simulink model "projetoRobotica"  (R2015a)
settings: Solver=ode1  StartTime=0.0  StopTime=inf  FixedStep=0.001  RelTol=1e-3
undefined symbols (not defined in the file or in its folder): qc_get_step_size
libraries: simulink x37, simulink_extras x12, quarc_library x8, instrumentlib x1
settings Model: SimulationMode=external  ExtModeTrigDuration=10000  Creator=CFulford  LastModifiedBy=RAS
settings SolverCC: PositivePriorityOrder=on
settings DataIOCC: LimitDataPoints=off  MaxDataPoints=10000  SignalLoggingSaveFormat=ModelDataLogs
settings OptimizationCC: ExpressionDepthLimit=2147483647  InitFltsAndDblsToZero=on
settings DebuggingCC: AlgebraicLoopMsg=none  SaveWithParameterizedLinksMsg=none  UnderspecifiedInitializationDetection=Classic  MergeDetectMultiDrivingBlocksExec=none  SolverPrmCheckMsg=warning  FcnCallInpInsideContextMsg=UseLocalSettings  StateNameClashWarn=warning
settings SFSimCC: SimParseCustomCode=off
settings RTWCC: SystemTargetFile=quarc_win64.tlc  TemplateMakefile=quarc_default_tmf  Description=QUARC Win64 Target
settings STFCustomTargetCC: TargetLibSuffix=.lib  TargetPreCompLibLocation=C:\PROGRA~3\QUARC\lib\2015a\win64\release  GenerateSampleERTMain=off  ConcurrentExecutionCompliant=on  GeneratePreprocessorConditionals=Disable all  CombineOutputUpdateFcns=on  ERTCustomFileBanners=off  SupportNonInlinedSFcns=on  SupportVariableSizeSignals=off  MATLABClassNameForMDSCustomization=Simulink.SoftwareTarget.GRTCustomization  CPPClassGenCompliant=on  SystemTargetFile=quarc_win64.tlc
settings GRTTargetCC: TargetPreCompLibLocation=C:\PROGRA~3\QUARC\lib\2015a\win64\release  ParMdlRefBuildCompliant=off  CompOptLevelCompliant=off  MatFileLogging=off  ExtMode=on  ExtModeMexFile=quarc_comm

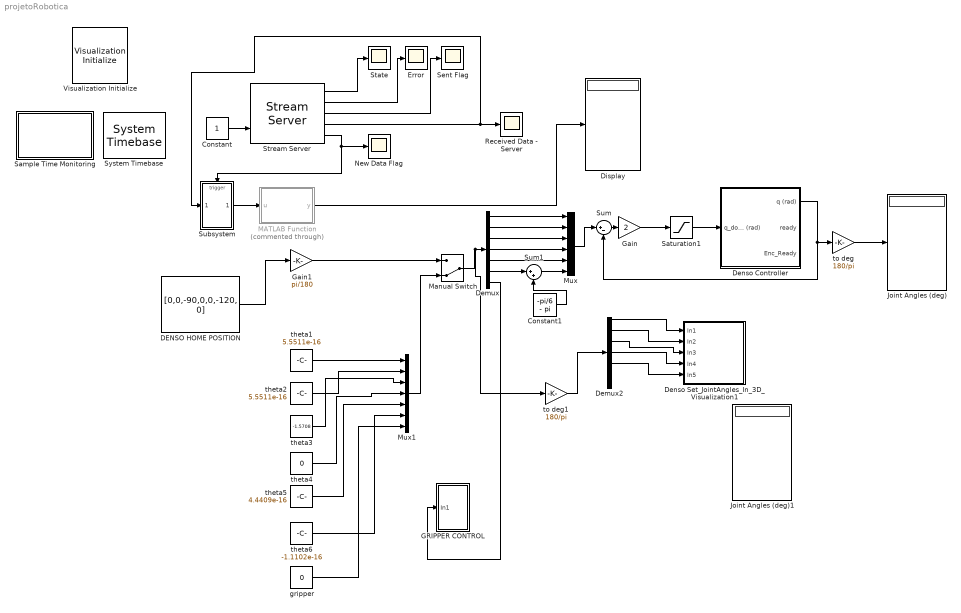
== system projetoRobotica ==
  Constant : Constant
  Constant1 : Constant  Value=-pi/6 - pi
  DENSO HOME POSITION : Constant  Value=[0,0,-90,0,0,-120, 0]  OutDataTypeStr=double  SampleTime=-1
  Demux : Demux  Outputs=7
  Demux2 : Demux  Outputs=7
  Denso Set_JointAngles_In_3D_Visualization1 : Subsystem
  Denso Controller : Subsystem
  Display : Display
  Error : Scope
      settings: SaveName=ScopeData6
  GRIPPER CONTROL : Subsystem
  Gain : Gain  Gain=2
  Gain1 : Gain  Gain=pi/180
  Joint Angles (deg) : Display
      settings: Decimation=100
  Joint Angles (deg)1 : Display
      settings: Decimation=100
  MATLAB Function : MATLAB Function  Commented=through  TreatAsAtomicUnit=on
  Manual Switch : ManualSwitch  CurrentSetting=0
  Mux : Mux  Inputs=6
  Mux1 : Mux  Inputs=7
  New Data Flag : Scope
      settings: SaveName=ScopeData7
  Received Data - Server : Scope
      settings: YMin=-0.2  YMax=1.2  SaveName=ScopeData8
  Sample Time Monitoring : Subsystem
  Saturation1 : Saturate  UpperLimit=200*pi/180  LowerLimit=-200*pi/180  OutDataTypeStr=double
  Sent Flag : Scope
      settings: SaveName=ScopeData5
  State : Scope
      settings: YMin=0  YMax=2
  Stream Server : quarc_library/Communications/Basic/Stream Server  uri_source=Specify via dialog (do not evaluate)  uri=tcpip://localhost:17001  apply_uri_to_all_configs=on  send_buffer_size=1460  receive_buffer_size=1460  byte_order=little endian (Intel - LSB first)  optimization=Minimum latency  implementation=Use non-blocking I/O  send_options=Send most recent data  receive_options=Receive most recent data  send_fifo_size=1000  receive_fifo_size=1000  send_priority=0  receive_priority=0  default_value=[0, 0, -pi/2, 0, 0, 0, 0]  send_dimensions=off  receive_dimensions=off  max_dimensions=-1  sample_time=qc_get_step_size  active=on  data_type=double  type_expr=BusObject
      settings: AttributesFormatString="\"tcpip://localhost:17001\""
  Subsystem : Subsystem
  Sum : Sum  Inputs=|+-
  Sum1 : Sum  Inputs=|++
  System Timebase : quarc_library/Advanced/Timing/System Timebase  stop_on_overrun=off
  Visualization Initialize : quarc_library/User Interface/Visualization/Visualization Initialize  object_name=kinect_direct_kinematics_3_angles_3D_Visualization  scene_file=kinect_direct_kinematics_3_angles_3D_Visualization.xml  uri={'normal','';'Configuration','shmem://%m:2';}  apply_uri_to_all_configs=off  server_send_size=1000000  server_receive_size=1000  derive_from_server=on  client_send_size=1000  client_receive_size=1000000  variables=[ 31 41 51 61 71 ]  initial_values=single([ 0 0 0 0 0 0 0 -1.5708 0 0 0 0 0 0 0 ])  open_on_start=on  close_on_stop=on
      settings: AttributesFormatString=%<object_name>
  gripper : Constant  Value=0
  theta1 : Constant  Value=5.5511e-16
  theta2 : Constant  Value=5.5511e-16
  theta3 : Constant  Value=-1.5708
  theta4 : Constant  Value=0
  theta5 : Constant  Value=4.4409e-16
  theta6 : Constant  Value=-1.1102e-16
  to deg : Gain  Gain=180/pi  OutDataTypeStr=single
  to deg1 : Gain  Gain=180/pi  ParamDataTypeStr=double  OutDataTypeStr=single
  wires:
  Stream Server/1 -> State/1
  Stream Server/2 -> Error/1
  Constant/1 -> Stream Server/2
  Stream Server/3 -> Sent Flag/1
  Stream Server/5 -> New Data Flag/1, Subsystem/Trigger
  Stream Server/4 -> Subsystem/1(In1), Received Data - Server/1
  to deg/1 -> Joint Angles (deg)/1
  Sum/1 -> Gain/1
  Gain/1 -> Saturation1/1
  Denso Controller/1(q (rad)) -> to deg/1, Sum/2
  Saturation1/1 -> Denso Controller/1(q_dot_cmd (rad))
  Subsystem/1(Out1) -> MATLAB Function/1(u)
  DENSO HOME POSITION/1 -> Gain1/1
  Demux2/5 -> Denso Set_JointAngles_In_3D_Visualization1/5(In5)
  Demux2/4 -> Denso Set_JointAngles_In_3D_Visualization1/4(In4)
  Demux2/2 -> Denso Set_JointAngles_In_3D_Visualization1/2(In2)
  Demux2/3 -> Denso Set_JointAngles_In_3D_Visualization1/3(In3)
  Demux2/1 -> Denso Set_JointAngles_In_3D_Visualization1/1(In1)
  to deg1/1 -> Demux2/1
  Manual Switch/1 -> to deg1/1, Demux/1
  Mux/1 -> Sum/1
  Demux/1 -> Mux/1
  Demux/2 -> Mux/2
  Demux/3 -> Mux/3
  Demux/4 -> Mux/4
  Demux/5 -> Mux/5
  Demux/7 -> GRIPPER CONTROL/1(In1)
  MATLAB Function/1(y) -> Display/1
  Demux/6 -> Sum1/1
  Sum1/1 -> Mux/6
  Constant1/1 -> Sum1/2
  theta1/1 -> Mux1/1
  theta2/1 -> Mux1/2
  theta4/1 -> Mux1/4
  theta5/1 -> Mux1/5
  Gain1/1 -> Manual Switch/1
  theta3/1 -> Mux1/3
  theta6/1 -> Mux1/6
  gripper/1 -> Mux1/7
  Mux1/1 -> Manual Switch/2

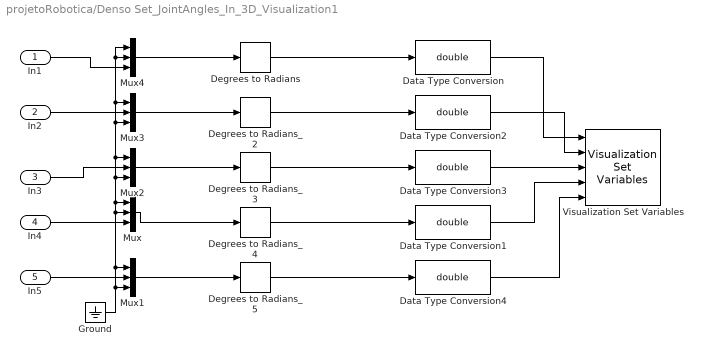
== system projetoRobotica/Denso Set_JointAngles_In_3D_Visualization1 ==
  In1 : Inport
  In2 : Inport  Port=2
  In3 : Inport  Port=3
  In4 : Inport  Port=4
  In5 : Inport  Port=5
  Data Type Conversion{,1..4} (5 alike) : DataTypeConversion  OutDataTypeStr=double
  Degrees to Radians : simulink_extras/Transformations/Degrees to Radians
  Degrees to Radians_{2..5} (4 alike) : simulink_extras/Transformations/Degrees to Radians
  Ground : Ground
  Mux{,1..4} (5 alike) : Mux  Inputs=3
  Visualization Set Variables : quarc_library/User Interface/Visualization/Visualization Set Variables  object_name=kinect_direct_kinematics_3_angles_3D_Visualization  offset=[ 0 3 6 9 12 ]  data_type=[ 0 0 0 0 0 ]  length=[ 3 3 3 3 3 ]  sample_time=visualization_get_frame_period  actor_name={'actor.Denso_Link1/Orientation';'actor.Denso_Link2/Orientation';'actor.Denso_Link3/Orientation';'actor.Denso_Link4/Orientation';'actor.Denso_Link5/Orientation'}
      settings: AttributesFormatString=(%<object_name>)
  wires:
  In3/1 -> Mux2/2
  Ground/1 -> Mux1/1, Mux/2, Mux/1, Mux2/1, Mux3/3, Mux3/1, Mux4/2, Mux4/1, Mux2/3, Mux1/3
  Data Type Conversion4/1 -> Visualization Set Variables/5
  Data Type Conversion1/1 -> Visualization Set Variables/4
  Data Type Conversion3/1 -> Visualization Set Variables/3
  Data Type Conversion2/1 -> Visualization Set Variables/2
  Data Type Conversion/1 -> Visualization Set Variables/1
  Mux2/1 -> Degrees to Radians_3/1
  Degrees to Radians_5/1 -> Data Type Conversion4/1
  Mux1/1 -> Degrees to Radians_5/1
  In5/1 -> Mux1/2
  Degrees to Radians_4/1 -> Data Type Conversion1/1
  Mux/1 -> Degrees to Radians_4/1
  In4/1 -> Mux/3
  Degrees to Radians_3/1 -> Data Type Conversion3/1
  In2/1 -> Mux3/2
  Mux3/1 -> Degrees to Radians_2/1
  Degrees to Radians_2/1 -> Data Type Conversion2/1
  Degrees to Radians/1 -> Data Type Conversion/1
  Mux4/1 -> Degrees to Radians/1
  In1/1 -> Mux4/3

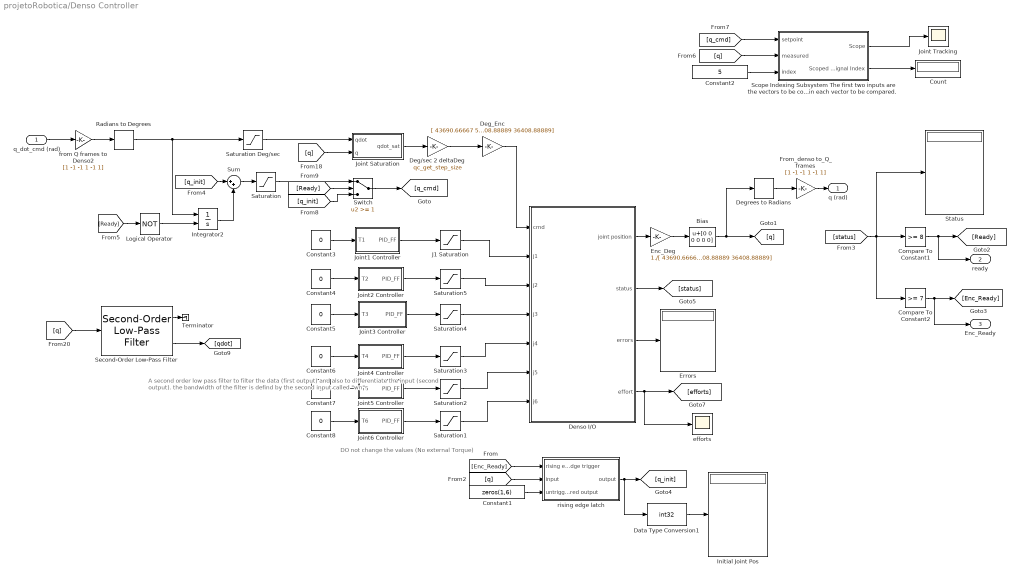
== system projetoRobotica/Denso Controller ==
  note: DO not change the values (No external Torque)
  note: A second order low pass filter to filter the data (first output) and also to differentiate
      |  the input (second output). the bandwidth of the filter is defind by the second input called "wn".
  q_dot_cmd (rad) : Inport
  Bias : Bias  Bias=[0 0 0 0 0 0]
  Compare To Constant1 : simulink/Logic and Bit Operations/Compare To Constant  relop=>=  const=8  OutDataTypeStr=uint8  ZeroCross=off
  Compare To Constant2 : simulink/Logic and Bit Operations/Compare To Constant  relop=>=  const=7  OutDataTypeStr=uint8  ZeroCross=off
  Constant1 : Constant  Value=zeros(1,6)
  Constant2 : Constant  Value=5
  Constant{3..8} (6 alike) : Constant  Value=0
  Count : Display
      settings: Decimation=100
  Data Type Conversion1 : DataTypeConversion  OutDataTypeStr=int32
  Deg/sec 2 deltaDeg : Gain  Gain=qc_get_step_size
  Deg_Enc : Gain  Gain=[ 43690.66667 58254.22222 43690.66667 36408.88889 36408.88889 36408.88889]
  Degrees to Radians : simulink_extras/Transformations/Degrees to Radians
  Denso I/O : Subsystem
  Enc_Deg : Gain  Gain=1./[ 43690.66667 58254.22222 43690.66667 36408.88889 36408.88889 36408.88889]
  Errors : Display
      settings: Decimation=100
  From_denso to_Q_frames : Gain  Gain=[1 -1 -1 1 -1 1]
  Initial Joint Pos : Display
      settings: Decimation=100
  Integrator2 : Integrator  ExternalReset=level
  J1 Saturation : Saturate  UpperLimit=3.7  LowerLimit=-3.7
  Joint Saturation : Subsystem
  Joint Tracking : Scope
      settings: TimeRange=2  YMin=93  YMax=100.5
  Joint1 Controller : Subsystem
  Joint2 Controller : Subsystem
  Joint3 Controller : Subsystem
  Joint4 Controller : Subsystem
  Joint5 Controller : Subsystem
  Joint6 Controller : Subsystem
  Logical Operator : Logic  Operator=NOT  AllPortsSameDT=off  OutDataTypeStr=boolean
  Radians to Degrees : simulink_extras/Transformations/Radians to Degrees
  Saturation : Saturate  UpperLimit=[160 65 162 162 100 365]  LowerLimit=-[160 122 20 162 100 365]
  Saturation Deg/sec : Saturate  UpperLimit="1e3*[1.1444    0.8583    1.1444    1.3733    1.3733    1.3733]"  LowerLimit="-1e3*[1.1444    0.8583    1.1444    1.3733    1.3733    1.3733]"
  Saturation{1..5} (5 alike) : Saturate  UpperLimit=3.7  LowerLimit=-3.7
  Scope Indexing Subsystem The first two inputs are the vectors to be compared. The third input is an index to define the elements in each vector to be compared. : Subsystem
  Second-Order Low-Pass Filter : quarc_library/Continuous/Second-Order Low-Pass Filter  params_source=Internal (dialog parameters)  input_width=60  input_zeta=1  input_init=0
  Status : Display
      settings: Decimation=100
  Sum : Sum  Inputs=|++
  Switch : Switch  Threshold=1
  Terminator : Terminator
  efforts : Scope
      settings: TimeRange=2  YMin=-4.5  YMax=0.5  SaveName=ScopeData3
  from Q frames to Denso2 : Gain  Gain=[1 -1 -1 1 -1 1]
  rising edge latch : Subsystem
  q (rad) : Outport
  ready : Outport  Port=2
  Enc_Ready : Outport  Port=3
  wires:
  Denso I/O/1(joint position) -> Enc_Deg/1
  Enc_Deg/1 -> Bias/1
  Joint2 Controller/1(PID_FF) -> Saturation5/1
  Joint3 Controller/1(PID_FF) -> Saturation4/1
  Joint1 Controller/1(PID_FF) -> J1 Saturation/1
  [Enc_Ready] -> rising edge latch/1(rising edge trigger)
  Compare To Constant1/1 -> ready/1, [Ready]
  [q] -> rising edge latch/2(input)
  rising edge latch/1(output) -> [q_init], Data Type Conversion1/1
  Constant1/1 -> rising edge latch/3(untriggered output)
  Denso I/O/4(effort) -> efforts/1, [efforts]
  Scope Indexing Subsystem The first two inputs are the vectors to be compared. The third input is an index to define the elements in each vector to be compared./2(Scoped Signal Index) -> Count/1
  Constant2/1 -> Scope Indexing Subsystem The first two inputs are the vectors to be compared. The third input is an index to define the elements in each vector to be compared./3(index)
  Compare To Constant2/1 -> Enc_Ready/1, [Enc_Ready]
  Denso I/O/2(status) -> [status]
  [status] -> Compare To Constant2/1, Status/1, Compare To Constant1/1
  [q_cmd] -> Scope Indexing Subsystem The first two inputs are the vectors to be compared. The third input is an index to define the elements in each vector to be compared./1(setpoint)
  [q] -> Scope Indexing Subsystem The first two inputs are the vectors to be compared. The third input is an index to define the elements in each vector to be compared./2(measured)
  [Ready] -> Logical Operator/1
  Logical Operator/1 -> Integrator2/2
  q_dot_cmd (rad)/1 -> from Q frames to Denso2/1
  Bias/1 -> Degrees to Radians/1, [q]
  Denso I/O/3(errors) -> Errors/1
  Degrees to Radians/1 -> From_denso to_Q_frames/1
  Deg/sec 2 deltaDeg/1 -> Deg_Enc/1
  From_denso to_Q_frames/1 -> q (rad)/1
  Joint4 Controller/1(PID_FF) -> Saturation3/1
  Joint5 Controller/1(PID_FF) -> Saturation2/1
  Joint6 Controller/1(PID_FF) -> Saturation1/1
  Saturation Deg/sec/1 -> Joint Saturation/1(qdot)
  [q] -> Joint Saturation/2(q)
  from Q frames to Denso2/1 -> Radians to Degrees/1
  Scope Indexing Subsystem The first two inputs are the vectors to be compared. The third input is an index to define the elements in each vector to be compared./1(Scope) -> Joint Tracking/1
  Data Type Conversion1/1 -> Initial Joint Pos/1
  Joint Saturation/1(qdot_sat) -> Deg/sec 2 deltaDeg/1
  [Ready] -> Switch/2
  Sum/1 -> Saturation/1
  Switch/1 -> [q_cmd]
  [q_init] -> Switch/3
  [q_init] -> Sum/1
  Integrator2/1 -> Sum/2
  Saturation/1 -> Switch/1
  Radians to Degrees/1 -> Integrator2/1, Saturation Deg/sec/1
  Deg_Enc/1 -> Denso I/O/1(cmd)
  Constant3/1 -> Joint1 Controller/1(T1)
  Constant4/1 -> Joint2 Controller/1(T2)
  Constant5/1 -> Joint3 Controller/1(T3)
  Constant6/1 -> Joint4 Controller/1(T4)
  Constant7/1 -> Joint5 Controller/1(T5)
  Constant8/1 -> Joint6 Controller/1(T6)
  Saturation4/1 -> Denso I/O/4(j3)
  Saturation5/1 -> Denso I/O/3(j2)
  Saturation3/1 -> Denso I/O/5(j4)
  J1 Saturation/1 -> Denso I/O/2(j1)
  Saturation2/1 -> Denso I/O/6(j5)
  Saturation1/1 -> Denso I/O/7(j6)
  [q] -> Second-Order Low-Pass Filter/1
  Second-Order Low-Pass Filter/2 -> [qdot]
  Second-Order Low-Pass Filter/1 -> Terminator/1

== system projetoRobotica/GRIPPER CONTROL ==
  note: Note: Always start with 1 when power up the gripper
  note: 1: Enable
      | 2: Predefined Close
      | 3: Predefined Open
      | 4: Custom Operation (Adjust Speed and Angle)
  In1 : Inport
  Communication_OK : Display
  Constant10 : Constant
  Constant82 : Constant  Value=4
  Constant9 : Constant
  Error1 : Display
  Manual Switch3 : ManualSwitch
  RobotiQ Gripper Control : Subsystem
  Slider Gain : simulink/Math Operations/Slider Gain  low=0  gain=0.85  high=1
  Slider Gain1 : simulink/Math Operations/Slider Gain  low=0  gain=1  high=1
  wires:
  Constant82/1 -> RobotiQ Gripper Control/1(Task)
  RobotiQ Gripper Control/1(Comm_OK) -> Communication_OK/1
  RobotiQ Gripper Control/2(Error) -> Error1/1
  Slider Gain1/1 -> RobotiQ Gripper Control/3("Speed (0: Minimum Speed, 1: Maximum Speed)")
  Constant10/1 -> Slider Gain1/1
  Constant9/1 -> Slider Gain/1
  Slider Gain/1 -> Manual Switch3/2
  Manual Switch3/1 -> RobotiQ Gripper Control/2("Angle (0: Full Open, 1: Full Close")
  In1/1 -> Manual Switch3/1

== system projetoRobotica/Sample Time Monitoring ==
  Clock : Clock
  Memory : Memory
  Running Time : Scope
      settings: TimeRange=2  YMin=0.00515  YMax=0.006  SaveName=ScopeData2
  Sample Time : quarc_library/Sources/Time/Sample Time  Priority=-99  sample_time=qc_get_step_size
  "Sample Time " : Scope
      settings: TimeRange=2  YMin=0  YMax=0.005  SaveName=ScopeData4
  Sum1 : Sum  Inputs=|++
  Sum2 : Sum  Inputs=|+-
  wires:
  Sample Time/1 -> "Sample Time "/1, Sum1/1
  Clock/1 -> Sum2/2
  Sum2/1 -> Running Time/1
  Sum1/1 -> Sum2/1, Memory/1
  Memory/1 -> Sum1/2

== system projetoRobotica/Subsystem ==
  note: J1
  note: J2
  note: J3
  note: J4
  note: J5
  note: J6
  note: Gripper
  In1 : Inport
  Trigger : TriggerPort  PortDimensions=1
  Demux : Demux  Outputs=7
  Demux1 : Demux  Outputs=6
  Denso Set_JointAngles_In_3D_Visualization : Subsystem
  Gain : Gain  Commented=through  Gain=-1
  Gain1 : Gain  Commented=through  Gain=-1
  Gain2 : Gain  Commented=through  Gain=-1
  Joint Angles (deg)1 : Display
      settings: Decimation=100
  Mux2 : Mux  Inputs=7
  TCP/IP Send : instrumentlib/TCP//IP Send  Host=localhost  Port=3142  EnableBlockingMode=on  Timeout=10  ByteOrder=LittleEndian
  to deg : Gain  Gain=180/pi  ParamDataTypeStr=double  OutDataTypeStr=single
  Out1 : Outport
  wires:
  Demux/3 -> Gain/1
  Demux1/5 -> Denso Set_JointAngles_In_3D_Visualization/5(In5)
  Demux1/4 -> Denso Set_JointAngles_In_3D_Visualization/4(In4)
  Demux1/2 -> Denso Set_JointAngles_In_3D_Visualization/2(In2)
  Demux1/3 -> Denso Set_JointAngles_In_3D_Visualization/3(In3)
  Demux/6 -> Mux2/6
  Mux2/1 -> Out1/1, to deg/1, TCP/IP Send/1, Joint Angles (deg)1/1
  Demux1/1 -> Denso Set_JointAngles_In_3D_Visualization/1(In1)
  In1/1 -> Demux/1
  Demux/5 -> Gain2/1
  Demux/2 -> Gain1/1
  Demux/1 -> Mux2/1
  Demux/4 -> Mux2/4
  Gain/1 -> Mux2/3
  to deg/1 -> Demux1/1
  Gain1/1 -> Mux2/2
  Gain2/1 -> Mux2/5
  Demux/7 -> Mux2/7

== system projetoRobotica/Denso Controller/Denso I//O ==
  cmd : Inport
  j1 : Inport  Port=2
  j2 : Inport  Port=3
  j3 : Inport  Port=4
  j4 : Inport  Port=5
  j5 : Inport  Port=6
  j6 : Inport  Port=7
  Denso Read : S-Function  FunctionName=denso_read_block  Parameters=uri  mask(Denso Read){uri=udp://192.168.0.1:1000}
      mask help: Initializes a connection to the Denso robot controller and reads the robot joint positions and state.
      mask init:
      | commands = { ...
      |     'port_label(''output'', 1, ''denso'');', ...
      |     'port_label(''output'', 2, ''position'');', ...
      |     'port_label(''output'', 3, ''effort'');', ...
      |     'port_label(''output'', 4, ''status'');' ...
      |     'port_label(''output'', 5, ''errors'');' ...
      | };
      | 
      | qc_set_display('Denso Read', commands);
      mask Display:
      | patch([0.98591 0.98591 0.62618 0.59072 0.56147   0.536   0.536  0.5441 0.56912 0.59207 0.60881 0.62276 0.63527 0.64364  0.6485  0.6485 0.64706 0.64499 0.63662 0.62411 0.61232 0.59837 0.58307 0.56147   0.536   0.536  0.5441  0.5747 0.60953 0.63662 0.67001  0.7034 0.72851 0.75425 0.77927 0.80294 0.82454 0.84119 0.85865 0.87395 0.88574 0.89339  0.8969 0.89969 0.89969 0.89267  0.8816 0.87044 0.85649  0.8384 0.81824 0.80294 0.78764 0.77513 0.76676 0.75776 0.76397 0.77513 0.79178 0.80987 0.82796 0.84326 0.86207 0.98528],[0.18689 0.05522 0.05522 0.05171 0.05171    0.05 0.18338 0.18338 0.19148 0.20435 0.22298 0.24863 0.28589 0.33125 0.38138 0.55139 0.59801 0.63761 0.68189 0.72149 0.74939 0.76694 0.77855 0.79367 0.79952 0.92768 0.92768 0.92768 0.92417 0.92066 0.91364  0.9032 0.89384 0.88106 0.86594 0.85073 0.82634 0.80537 0.77855 0.74363 0.70403 0.65858 0.61079 0.59099 0.41513 0.37202 0.31847 0.29048 0.25556 0.23342  0.2102 0.19382 0.18221 0.17285 0.16943 0.16124  0.1589 0.16241 0.16709 0.17168  0.1787 0.18221 0.18689 0.18689],[0.9,0.90,0.91])
      | patch([0.536 0.52601 0.46823 0.44528 0.41603 0.39101 0.35555 0.33116 0.31451 0.29291  0.2804 0.26717 0.25322 0.23999 0.22406 0.20732 0.19337 0.17528 0.15935 0.14396 0.13217 0.11759 0.10922 0.10085 0.09671 0.09392 0.09041 0.08906 0.08906 0.09464  0.0995 0.10778 0.11894 0.13145 0.14675 0.16349 0.17672 0.19409 0.20732 0.22406 0.23999 0.26159 0.27833 0.29849 0.31793 0.33602 0.35411 0.37085 0.39245 0.41603   0.536   0.536 0.53159 0.46409   0.446 0.42026 0.39587 0.37571 0.36113 0.34925 0.34088 0.33809 0.33809 0.34088 0.34583 0.35627 0.36392 0.38129 0.39587 0.41117 0.42719 0.44672  0.4676 0.48353 0.48353 0.52394   0.536],[0.05 0.04829 0.04712 0.04712 0.04829 0.05063 0.05405 0.05873 0.06107 0.06692 0.07043 0.07619 0.08087 0.08672 0.09482 0.10652 0.11696 0.13325  0.1508 0.17168 0.19499 0.22415 0.25439 0.28472 0.31379 0.35456 0.38489 0.41513 0.58055 0.63878 0.68774 0.72149 0.75641 0.78089 0.80537 0.82859 0.84029 0.85658 0.86594 0.87404  0.8834 0.89267 0.90086 0.90788 0.91247 0.91832 0.92066   0.923 0.92651 0.92768 0.92768 0.79952 0.79952 0.79952 0.79718 0.78899 0.77153 0.75056 0.72149 0.68072 0.62249  0.5549 0.41396 0.37085 0.33242 0.28121 0.25205 0.22181 0.20552 0.19499 0.18572 0.18221 0.17753 0.17636 0.17753  0.1787  0.1787],[0.9,0.90,0.91])
      | disp('Denso Read');
      | port_label('output', 1, 'denso');
      | port_label('output', 2, 'position');
      | port_label('output', 3, 'effort');
      | port_label('output', 4, 'status');
      | port_label('output', 5, 'errors');
  Denso Write : S-Function  FunctionName=denso_write_block  Parameters=velocity_mode  mask(Denso Write){velocity_mode=on}
      mask prompts: velocity_mode "Velocity mode"
      mask help: Sends joint commands and controller gains to the Denso robot.
      mask init:
      | commands = { ...
      |     'port_label(''input'', 1, ''denso'');', ...
      |     'port_label(''input'', 2, ''command'');', ...
      |     'port_label(''input'', 3, ''J1 gains'');', ...
      |     'port_label(''input'', 4, ''J2 gains'');' ...
      |     'port_label(''input'', 5, ''J3 gains'');' ...
      |     'port_label(''input'', 6, ''J4 gains'');' ...
      |     'port_label(''input'', 7, ''J5 gains'');' ...
      |     'port_label(''input'', 8, ''J6 gains'');' ...
      | };
      | 
      | qc_set_display('Denso Write', commands);
      mask Display:
      | patch([0.98591 0.98591 0.62618 0.59072 0.56147   0.536   0.536  0.5441 0.56912 0.59207 0.60881 0.62276 0.63527 0.64364  0.6485  0.6485 0.64706 0.64499 0.63662 0.62411 0.61232 0.59837 0.58307 0.56147   0.536   0.536  0.5441  0.5747 0.60953 0.63662 0.67001  0.7034 0.72851 0.75425 0.77927 0.80294 0.82454 0.84119 0.85865 0.87395 0.88574 0.89339  0.8969 0.89969 0.89969 0.89267  0.8816 0.87044 0.85649  0.8384 0.81824 0.80294 0.78764 0.77513 0.76676 0.75776 0.76397 0.77513 0.79178 0.80987 0.82796 0.84326 0.86207 0.98528],[0.18689 0.05522 0.05522 0.05171 0.05171    0.05 0.18338 0.18338 0.19148 0.20435 0.22298 0.24863 0.28589 0.33125 0.38138 0.55139 0.59801 0.63761 0.68189 0.72149 0.74939 0.76694 0.77855 0.79367 0.79952 0.92768 0.92768 0.92768 0.92417 0.92066 0.91364  0.9032 0.89384 0.88106 0.86594 0.85073 0.82634 0.80537 0.77855 0.74363 0.70403 0.65858 0.61079 0.59099 0.41513 0.37202 0.31847 0.29048 0.25556 0.23342  0.2102 0.19382 0.18221 0.17285 0.16943 0.16124  0.1589 0.16241 0.16709 0.17168  0.1787 0.18221 0.18689 0.18689],[0.9,0.90,0.91])
      | patch([0.536 0.52601 0.46823 0.44528 0.41603 0.39101 0.35555 0.33116 0.31451 0.29291  0.2804 0.26717 0.25322 0.23999 0.22406 0.20732 0.19337 0.17528 0.15935 0.14396 0.13217 0.11759 0.10922 0.10085 0.09671 0.09392 0.09041 0.08906 0.08906 0.09464  0.0995 0.10778 0.11894 0.13145 0.14675 0.16349 0.17672 0.19409 0.20732 0.22406 0.23999 0.26159 0.27833 0.29849 0.31793 0.33602 0.35411 0.37085 0.39245 0.41603   0.536   0.536 0.53159 0.46409   0.446 0.42026 0.39587 0.37571 0.36113 0.34925 0.34088 0.33809 0.33809 0.34088 0.34583 0.35627 0.36392 0.38129 0.39587 0.41117 0.42719 0.44672  0.4676 0.48353 0.48353 0.52394   0.536],[0.05 0.04829 0.04712 0.04712 0.04829 0.05063 0.05405 0.05873 0.06107 0.06692 0.07043 0.07619 0.08087 0.08672 0.09482 0.10652 0.11696 0.13325  0.1508 0.17168 0.19499 0.22415 0.25439 0.28472 0.31379 0.35456 0.38489 0.41513 0.58055 0.63878 0.68774 0.72149 0.75641 0.78089 0.80537 0.82859 0.84029 0.85658 0.86594 0.87404  0.8834 0.89267 0.90086 0.90788 0.91247 0.91832 0.92066   0.923 0.92651 0.92768 0.92768 0.79952 0.79952 0.79952 0.79718 0.78899 0.77153 0.75056 0.72149 0.68072 0.62249  0.5549 0.41396 0.37085 0.33242 0.28121 0.25205 0.22181 0.20552 0.19499 0.18572 0.18221 0.17753 0.17636 0.17753  0.1787  0.1787],[0.9,0.90,0.91])
      | disp('Denso Write');
      | port_label('input', 1, 'denso');
      | port_label('input', 2, 'command');
      | port_label('input', 3, 'J1 gains');
      | port_label('input', 4, 'J2 gains');
      | port_label('input', 5, 'J3 gains');
      | port_label('input', 6, 'J4 gains');
      | port_label('input', 7, 'J5 gains');
      | port_label('input', 8, 'J6 gains');
  joint position : Outport
  status : Outport  Port=2
  errors : Outport  Port=3
  effort : Outport  Port=4
  wires:
  j6/1 -> Denso Write/8
  j5/1 -> Denso Write/7
  j4/1 -> Denso Write/6
  j3/1 -> Denso Write/5
  j2/1 -> Denso Write/4
  Denso Read/5 -> errors/1
  Denso Read/4 -> status/1
  Denso Read/3 -> effort/1
  Denso Read/2 -> joint position/1
  Denso Read/1 -> Denso Write/1
  cmd/1 -> Denso Write/2
  j1/1 -> Denso Write/3

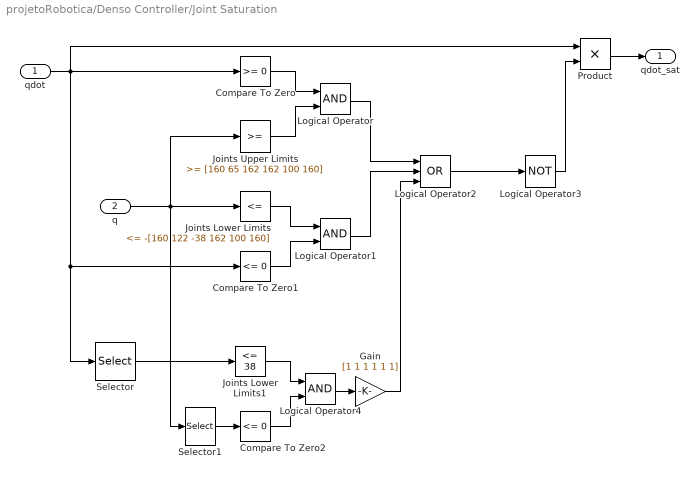
== system projetoRobotica/Denso Controller/Joint Saturation ==
  qdot : Inport
  q : Inport  Port=2
  Compare To Zero : simulink/Logic and Bit Operations/Compare To Zero  relop=>=  OutDataTypeStr=uint8  ZeroCross=off
  Compare To Zero1 : simulink/Logic and Bit Operations/Compare To Zero  relop=<=  OutDataTypeStr=uint8  ZeroCross=off
  Compare To Zero2 : simulink/Logic and Bit Operations/Compare To Zero  relop=<=  OutDataTypeStr=uint8  ZeroCross=off
  Gain : Gain  Gain=[1 1 1 1 1 1]
  Joints Lower Limits : simulink/Logic and Bit Operations/Compare To Constant  relop=<=  const=-[160 122 -38 162 100 160]  OutDataTypeStr=uint8  ZeroCross=off
  Joints Lower Limits1 : simulink/Logic and Bit Operations/Compare To Constant  relop=<=  const=38  OutDataTypeStr=uint8  ZeroCross=off
  Joints Upper Limits : simulink/Logic and Bit Operations/Compare To Constant  relop=>=  const=[160 65 162 162 100 160]  OutDataTypeStr=uint8  ZeroCross=off
  Logical Operator : Logic  AllPortsSameDT=off  OutDataTypeStr=boolean
  Logical Operator1 : Logic  AllPortsSameDT=off  OutDataTypeStr=boolean
  Logical Operator2 : Logic  Operator=OR  Inputs=3  AllPortsSameDT=off  OutDataTypeStr=boolean
  Logical Operator3 : Logic  Operator=NOT  AllPortsSameDT=off  OutDataTypeStr=boolean
  Logical Operator4 : Logic  AllPortsSameDT=off  OutDataTypeStr=boolean
  Product : Product  RndMeth=Zero
  Selector : Selector  InputPortWidth=6  Indices=3
  Selector1 : Selector  InputPortWidth=6  Indices=3
  qdot_sat : Outport
  wires:
  q/1 -> Joints Lower Limits/1, Joints Upper Limits/1, Selector1/1
  Logical Operator2/1 -> Logical Operator3/1
  Compare To Zero/1 -> Logical Operator/1
  Joints Upper Limits/1 -> Logical Operator/2
  Joints Lower Limits/1 -> Logical Operator1/1
  Compare To Zero1/1 -> Logical Operator1/2
  Logical Operator/1 -> Logical Operator2/1
  Logical Operator1/1 -> Logical Operator2/2
  qdot/1 -> Compare To Zero/1, Product/1, Compare To Zero1/1, Selector/1
  Logical Operator3/1 -> Product/2
  Product/1 -> qdot_sat/1
  Joints Lower Limits1/1 -> Logical Operator4/1
  Compare To Zero2/1 -> Logical Operator4/2
  Selector/1 -> Joints Lower Limits1/1
  Selector1/1 -> Compare To Zero2/1
  Logical Operator4/1 -> Gain/1
  Gain/1 -> Logical Operator2/3

== system projetoRobotica/Denso Controller/Joint1 Controller ==
  T1 : Inport
  Constant12 : Constant
  Constant6 : Constant  Value=[1 0.1 28 35]
  Gain : Gain  Gain=1/.38*120
  Gain3 : Gain  Gain="[1 1 1   1]"
  Mux2 : Mux
  Slider Gain : simulink/Math Operations/Slider Gain  low=0  gain=0.22  high=1
  Slider Gain1 : simulink/Math Operations/Slider Gain  low=0  gain=0.1  high=24
  Slider Gain2 : simulink/Math Operations/Slider Gain  low=0  gain=24  high=100
  Terminator_1 : Terminator
  PID_FF : Outport
  wires:
  Mux2/1 -> Gain3/1
  Constant12/1 -> Slider Gain/1, Slider Gain1/1, Slider Gain2/1
  Slider Gain/1 -> Mux2/1
  Slider Gain1/1 -> Mux2/2
  Slider Gain2/1 -> Mux2/3
  Gain3/1 -> PID_FF/1
  Constant6/1 -> Terminator_1/1
  T1/1 -> Gain/1
  Gain/1 -> Mux2/4

== system projetoRobotica/Denso Controller/Joint2 Controller ==
  T2 : Inport
  Constant12 : Constant
  Gain : Gain  Gain=1/.38*160
  Mux2 : Mux
  Slider Gain : simulink/Math Operations/Slider Gain  low=0  gain=0.1512  high=1
  Slider Gain1 : simulink/Math Operations/Slider Gain  low=0  gain=0.08  high=0.1
  Slider Gain2 : simulink/Math Operations/Slider Gain  low=0  gain=14.88  high=20
  PID_FF : Outport
  wires:
  Slider Gain2/1 -> Mux2/3
  Slider Gain1/1 -> Mux2/2
  Slider Gain/1 -> Mux2/1
  Constant12/1 -> Slider Gain1/1, Slider Gain2/1, Slider Gain/1
  Mux2/1 -> PID_FF/1
  Gain/1 -> Mux2/4
  T2/1 -> Gain/1

== system projetoRobotica/Denso Controller/Joint3 Controller ==
  T3 : Inport
  Constant12 : Constant
  Gain : Gain  Gain=1/.38*120
  Mux2 : Mux
  Slider Gain : simulink/Math Operations/Slider Gain  low=0  gain=0.19  high=0.4
  Slider Gain1 : simulink/Math Operations/Slider Gain  low=0  gain=0.3  high=0.5
  Slider Gain2 : simulink/Math Operations/Slider Gain  low=0  gain=10.8  high=18
  PID_FF : Outport
  wires:
  Mux2/1 -> PID_FF/1
  Constant12/1 -> Slider Gain/1, Slider Gain1/1, Slider Gain2/1
  Slider Gain/1 -> Mux2/1
  Slider Gain1/1 -> Mux2/2
  Slider Gain2/1 -> Mux2/3
  T3/1 -> Gain/1
  Gain/1 -> Mux2/4

== system projetoRobotica/Denso Controller/Joint4 Controller ==
  T4 : Inport
  Constant12 : Constant
  Gain : Gain  Gain=1/.22*100
  Mux2 : Mux
  Slider Gain : simulink/Math Operations/Slider Gain  low=0  gain=0.05  high=0.1
  Slider Gain1 : simulink/Math Operations/Slider Gain  low=0  gain=0.05  high=0.2
  Slider Gain2 : simulink/Math Operations/Slider Gain  low=0  gain=1.4  high=2
  PID_FF : Outport
  wires:
  Gain/1 -> Mux2/4
  Slider Gain2/1 -> Mux2/3
  Slider Gain1/1 -> Mux2/2
  Slider Gain/1 -> Mux2/1
  Constant12/1 -> Slider Gain1/1, Slider Gain2/1, Slider Gain/1
  Mux2/1 -> PID_FF/1
  T4/1 -> Gain/1

== system projetoRobotica/Denso Controller/Joint5 Controller ==
  T5 : Inport
  Constant12 : Constant
  Gain : Gain  Gain=1/.21*100
  Mux2 : Mux
  Slider Gain : simulink/Math Operations/Slider Gain  low=0  gain=0.182  high=0.2
  Slider Gain1 : simulink/Math Operations/Slider Gain  low=0  gain=0.087  high=0.2
  Slider Gain2 : simulink/Math Operations/Slider Gain  low=0  gain=4.25  high=5
  PID_FF : Outport
  wires:
  Mux2/1 -> PID_FF/1
  Constant12/1 -> Slider Gain/1, Slider Gain1/1, Slider Gain2/1
  Slider Gain/1 -> Mux2/1
  Slider Gain1/1 -> Mux2/2
  Slider Gain2/1 -> Mux2/3
  Gain/1 -> Mux2/4
  T5/1 -> Gain/1

== system projetoRobotica/Denso Controller/Joint6 Controller ==
  T6 : Inport
  Constant12 : Constant
  Gain : Gain  Gain=1/.21*100
  Mux2 : Mux
  Slider Gain : simulink/Math Operations/Slider Gain  low=0  gain=0.1  high=0.2
  Slider Gain1 : simulink/Math Operations/Slider Gain  low=0  gain=0.1  high=0.1
  Slider Gain2 : simulink/Math Operations/Slider Gain  low=0  gain=3  high=3
  PID_FF : Outport
  wires:
  Slider Gain2/1 -> Mux2/3
  Slider Gain1/1 -> Mux2/2
  Slider Gain/1 -> Mux2/1
  Constant12/1 -> Slider Gain1/1, Slider Gain2/1, Slider Gain/1
  Mux2/1 -> PID_FF/1
  Gain/1 -> Mux2/4
  T6/1 -> Gain/1

== system projetoRobotica/Denso Controller/Scope Indexing Subsystem The first two inputs are the vectors to be compared. The third input is an index to define the elements in each vector to be compared. ==
  setpoint : Inport
  measured : Inport  Port=2
  index : Inport  Port=3
  Dynamic Router : MATLAB Function  TreatAsAtomicUnit=on
  Dynamic Router1 : MATLAB Function  TreatAsAtomicUnit=on
  Mux2 : Mux  Inputs=2
  Scope : Outport
  Scoped Signal Index : Outport  Port=2
  wires:
  Dynamic Router/1(signal) -> Mux2/1
  Dynamic Router1/1(signal) -> Mux2/2
  index/1 -> Dynamic Router/2(index), Dynamic Router1/2(index), Scoped Signal Index/1
  setpoint/1 -> Dynamic Router/1(array)
  measured/1 -> Dynamic Router1/1(array)
  Mux2/1 -> Scope/1

== system projetoRobotica/Denso Controller/rising edge latch ==
  rising edge trigger : Inport
  input : Inport  Port=2
  untriggered output : Inport  Port=3
  Latch Input : Subsystem  TreatAsAtomicUnit=on
  Switch : Switch  Threshold=0.5
  output : Outport
  wires:
  untriggered output/1 -> Switch/3
  Switch/1 -> output/1
  Latch Input/1(Latch) -> Switch/1
  Latch Input/2(Executed) -> Switch/2
  input/1 -> Latch Input/1(Input)
  rising edge trigger/1 -> Latch Input/Trigger

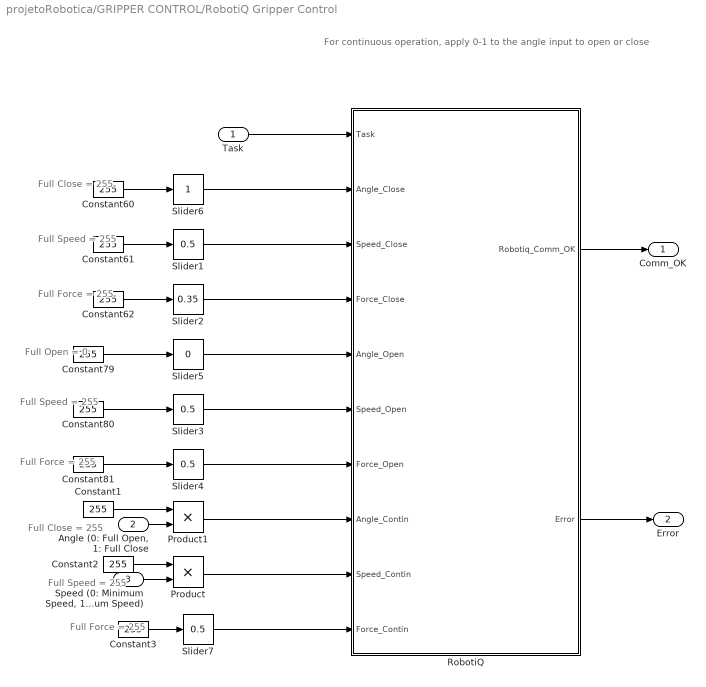
== system projetoRobotica/GRIPPER CONTROL/RobotiQ Gripper Control ==
  note: Full Close = 255
  note: Full Speed = 255
  note: Full Force = 255
  note: Full Open = 0
  note: Full Speed = 255
  note: Full Force = 255
  note: For continuous operation, apply 0-1 to the angle input to open or close
  note: Full Close = 255
  note: Full Speed = 255
  note: Full Force = 255
  Task : Inport
  "Angle (0: Full Open, 1: Full Close" : Inport  Port=2
  "Speed (0: Minimum Speed, 1: Maximum Speed)" : Inport  Port=3
  Constant{1..3,60..62,79..81} (9 alike) : Constant  Value=255
  Product : Product  RndMeth=Zero
  Product1 : Product  RndMeth=Zero
  RobotiQ : Subsystem
  Slider{1,3..4,7} (4 alike) : simulink/Math Operations/Slider Gain  low=0  gain=0.5  high=1
  Slider2 : simulink/Math Operations/Slider Gain  low=0  gain=0.35  high=1
  Slider5 : simulink/Math Operations/Slider Gain  low=0  gain=0  high=1
  Slider6 : simulink/Math Operations/Slider Gain  low=0  gain=1  high=1
  Comm_OK : Outport
  Error : Outport  Port=2
  wires:
  Constant62/1 -> Slider2/1
  Constant79/1 -> Slider5/1
  Constant80/1 -> Slider3/1
  Constant81/1 -> Slider4/1
  Slider2/1 -> RobotiQ/4(Force_Close)
  Slider3/1 -> RobotiQ/6(Speed_Open)
  Slider4/1 -> RobotiQ/7(Force_Open)
  Slider5/1 -> RobotiQ/5(Angle_Open)
  Task/1 -> RobotiQ/1(Task)
  RobotiQ/1(Robotiq_Comm_OK) -> Comm_OK/1
  "Angle (0: Full Open, 1: Full Close"/1 -> Product1/2
  "Speed (0: Minimum Speed, 1: Maximum Speed)"/1 -> Product/2
  RobotiQ/2(Error) -> Error/1
  Constant61/1 -> Slider1/1
  Slider1/1 -> RobotiQ/3(Speed_Close)
  Constant60/1 -> Slider6/1
  Slider6/1 -> RobotiQ/2(Angle_Close)
  Constant1/1 -> Product1/1
  Product1/1 -> RobotiQ/8(Angle_Contin)
  Constant2/1 -> Product/1
  Product/1 -> RobotiQ/9(Speed_Contin)
  Constant3/1 -> Slider7/1
  Slider7/1 -> RobotiQ/10(Force_Contin)

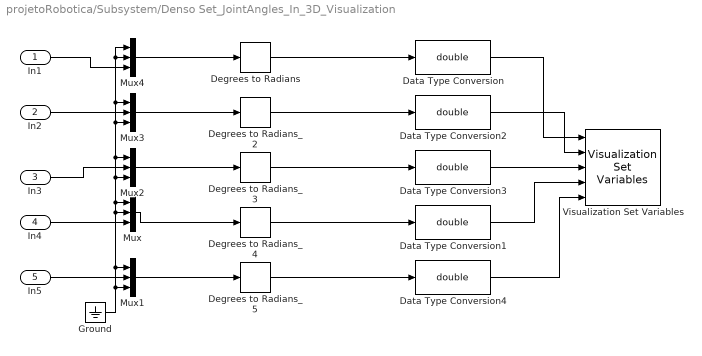
== system projetoRobotica/Subsystem/Denso Set_JointAngles_In_3D_Visualization ==
  In1 : Inport
  In2 : Inport  Port=2
  In3 : Inport  Port=3
  In4 : Inport  Port=4
  In5 : Inport  Port=5
  Data Type Conversion{,1..4} (5 alike) : DataTypeConversion  OutDataTypeStr=double
  Degrees to Radians : simulink_extras/Transformations/Degrees to Radians
  Degrees to Radians_{2..5} (4 alike) : simulink_extras/Transformations/Degrees to Radians
  Ground : Ground
  Mux{,1..4} (5 alike) : Mux  Inputs=3
  Visualization Set Variables : quarc_library/User Interface/Visualization/Visualization Set Variables  object_name=kinect_direct_kinematics_3_angles_3D_Visualization  offset=[ 0 3 6 9 12 ]  data_type=[ 0 0 0 0 0 ]  length=[ 3 3 3 3 3 ]  sample_time=visualization_get_frame_period  actor_name={'actor.Denso_Link1/Orientation';'actor.Denso_Link2/Orientation';'actor.Denso_Link3/Orientation';'actor.Denso_Link4/Orientation';'actor.Denso_Link5/Orientation'}
      settings: AttributesFormatString=(%<object_name>)
  wires:
  In1/1 -> Mux4/3
  Mux4/1 -> Degrees to Radians/1
  Degrees to Radians/1 -> Data Type Conversion/1
  Degrees to Radians_2/1 -> Data Type Conversion2/1
  Mux3/1 -> Degrees to Radians_2/1
  In2/1 -> Mux3/2
  Degrees to Radians_3/1 -> Data Type Conversion3/1
  In4/1 -> Mux/3
  Mux/1 -> Degrees to Radians_4/1
  Degrees to Radians_4/1 -> Data Type Conversion1/1
  In5/1 -> Mux1/2
  Mux1/1 -> Degrees to Radians_5/1
  Degrees to Radians_5/1 -> Data Type Conversion4/1
  Mux2/1 -> Degrees to Radians_3/1
  Data Type Conversion/1 -> Visualization Set Variables/1
  Data Type Conversion2/1 -> Visualization Set Variables/2
  Data Type Conversion3/1 -> Visualization Set Variables/3
  Data Type Conversion1/1 -> Visualization Set Variables/4
  Data Type Conversion4/1 -> Visualization Set Variables/5
  Ground/1 -> Mux1/3, Mux2/3, Mux4/1, Mux4/2, Mux3/1, Mux3/3, Mux2/1, Mux/1, Mux/2, Mux1/1
  In3/1 -> Mux2/2

== system projetoRobotica/Denso Controller/rising edge latch/Latch Input ==
  Input : Inport
  Trigger : TriggerPort
  Constant : Constant
  Latch : Outport
  Executed : Outport  Port=2
  wires:
  Constant/1 -> Executed/1
  Input/1 -> Latch/1

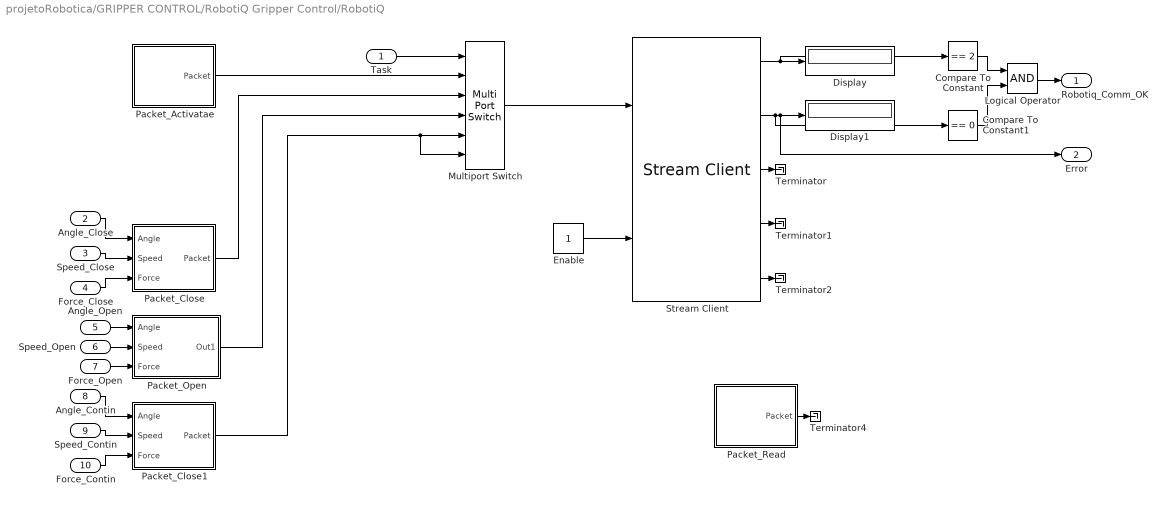
== system projetoRobotica/GRIPPER CONTROL/RobotiQ Gripper Control/RobotiQ ==
  Task : Inport
  Angle_Close : Inport  Port=2
  Speed_Close : Inport  Port=3
  Force_Close : Inport  Port=4
  Angle_Open : Inport  Port=5
  Speed_Open : Inport  Port=6
  Force_Open : Inport  Port=7
  Angle_Contin : Inport  Port=8
  Speed_Contin : Inport  Port=9
  Force_Contin : Inport  Port=10
  Compare To Constant : simulink/Logic and Bit Operations/Compare To Constant  relop===  const=2  OutDataTypeStr=uint8
  Compare To Constant1 : simulink/Logic and Bit Operations/Compare To Constant  relop===  const=0  OutDataTypeStr=uint8
  Display : Display
  Display1 : Display
  Enable : Constant
  Logical Operator : Logic  AllPortsSameDT=off  OutDataTypeStr=boolean
  Multiport Switch : MultiPortSwitch  Inputs=5  AllowDiffInputSizes=on
  Packet_Activatae : Subsystem
  Packet_Close : Subsystem
  Packet_Close1 : Subsystem
  Packet_Open : Subsystem
  Packet_Read : Subsystem
  Stream Client : quarc_library/Communications/Basic/Stream Client  uri_source=Specify via dialog (do not evaluate)  uri=tcpip://192.168.1.11:502  apply_uri_to_all_configs=on  send_buffer_size=1460  receive_buffer_size=1460  byte_order=little endian (Intel - LSB first)  optimization=Minimum latency  implementation=Use blocking I/O in a separate thread  send_options=Send most recent data  receive_options=Receive all data  send_fifo_size=1000  receive_fifo_size=1000  send_priority=0  receive_priority=0  default_value=zeros(12,1)  send_dimensions=off  receive_dimensions=off  max_dimensions=-1  sample_time=qc_get_step_size  active=on  data_type=uint8  type_expr=BusObject
      settings: AttributesFormatString="\"tcpip://192.168.1.11:502\""
  Terminator{,1..2,4} (4 alike) : Terminator
  Robotiq_Comm_OK : Outport
  Error : Outport  Port=2
  wires:
  Stream Client/1 -> Display/1, Compare To Constant/1
  Stream Client/2 -> Compare To Constant1/1, Display1/1, Error/1
  Enable/1 -> Stream Client/2
  Packet_Activatae/1(Packet) -> Multiport Switch/2
  Packet_Close/1(Packet) -> Multiport Switch/3
  Multiport Switch/1 -> Stream Client/1
  Compare To Constant/1 -> Logical Operator/1
  Compare To Constant1/1 -> Logical Operator/2
  Task/1 -> Multiport Switch/1
  Logical Operator/1 -> Robotiq_Comm_OK/1
  Angle_Close/1 -> Packet_Close/1(Angle)
  Speed_Close/1 -> Packet_Close/2(Speed)
  Force_Close/1 -> Packet_Close/3(Force)
  Stream Client/3 -> Terminator/1
  Stream Client/4 -> Terminator1/1
  Stream Client/5 -> Terminator2/1
  Speed_Open/1 -> Packet_Open/2(Speed)
  Force_Open/1 -> Packet_Open/3(Force)
  Angle_Open/1 -> Packet_Open/1(Angle)
  Packet_Open/1(Out1) -> Multiport Switch/4
  Packet_Read/1(Packet) -> Terminator4/1
  Angle_Contin/1 -> Packet_Close1/1(Angle)
  Speed_Contin/1 -> Packet_Close1/2(Speed)
  Force_Contin/1 -> Packet_Close1/3(Force)
  Packet_Close1/1(Packet) -> Multiport Switch/5, Multiport Switch/6

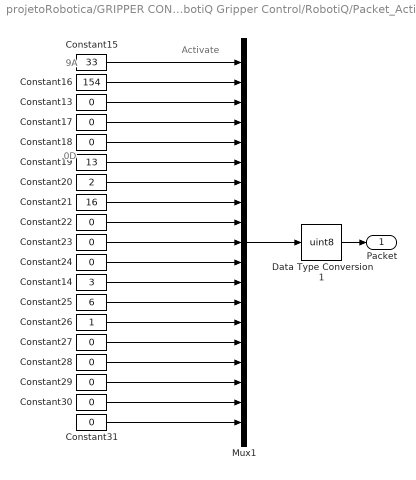
== system projetoRobotica/GRIPPER CONTROL/RobotiQ Gripper Control/RobotiQ/Packet_Activatae ==
  note: 9A
  note: 0D
  note: Activate
  Constant{13,17..18,22..24,27..31} (11 alike) : Constant  Value=0
  Constant14 : Constant  Value=3
  Constant15 : Constant  Value=33
  Constant16 : Constant  Value=154
  Constant19 : Constant  Value=13
  Constant20 : Constant  Value=2
  Constant21 : Constant  Value=16
  Constant25 : Constant  Value=6
  Constant26 : Constant
  Data Type Conversion1 : DataTypeConversion  OutDataTypeStr=uint8
  Mux1 : Mux  Inputs=19
  Packet : Outport
  wires:
  Mux1/1 -> Data Type Conversion1/1
  Constant13/1 -> Mux1/3
  Constant17/1 -> Mux1/4
  Constant18/1 -> Mux1/5
  Constant19/1 -> Mux1/6
  Constant20/1 -> Mux1/7
  Constant21/1 -> Mux1/8
  Constant22/1 -> Mux1/9
  Constant23/1 -> Mux1/10
  Constant24/1 -> Mux1/11
  Constant14/1 -> Mux1/12
  Constant15/1 -> Mux1/1
  Constant16/1 -> Mux1/2
  Constant25/1 -> Mux1/13
  Constant26/1 -> Mux1/14
  Constant27/1 -> Mux1/15
  Constant28/1 -> Mux1/16
  Constant29/1 -> Mux1/17
  Constant30/1 -> Mux1/18
  Constant31/1 -> Mux1/19
  Data Type Conversion1/1 -> Packet/1

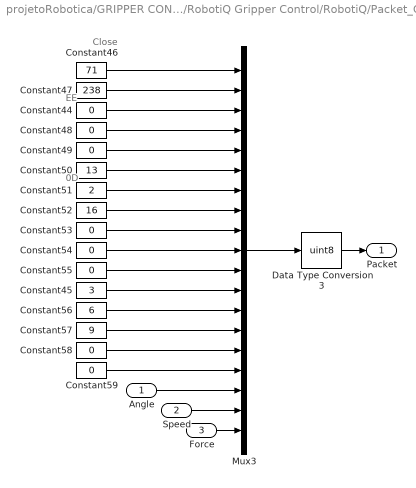
== system projetoRobotica/GRIPPER CONTROL/RobotiQ Gripper Control/RobotiQ/Packet_Close ==
  note: EE
  note: 0D
  note: Close
  Angle : Inport
  Speed : Inport  Port=2
  Force : Inport  Port=3
  Constant{44,48..49,53..55,58..59} (8 alike) : Constant  Value=0
  Constant45 : Constant  Value=3
  Constant46 : Constant  Value=71
  Constant47 : Constant  Value=238
  Constant50 : Constant  Value=13
  Constant51 : Constant  Value=2
  Constant52 : Constant  Value=16
  Constant56 : Constant  Value=6
  Constant57 : Constant  Value=9
  Data Type Conversion3 : DataTypeConversion  OutDataTypeStr=uint8
  Mux3 : Mux  Inputs=19
  Packet : Outport
  wires:
  Mux3/1 -> Data Type Conversion3/1
  Constant44/1 -> Mux3/3
  Constant48/1 -> Mux3/4
  Constant49/1 -> Mux3/5
  Constant50/1 -> Mux3/6
  Constant51/1 -> Mux3/7
  Constant52/1 -> Mux3/8
  Constant53/1 -> Mux3/9
  Constant54/1 -> Mux3/10
  Constant55/1 -> Mux3/11
  Constant45/1 -> Mux3/12
  Constant46/1 -> Mux3/1
  Constant47/1 -> Mux3/2
  Constant56/1 -> Mux3/13
  Constant57/1 -> Mux3/14
  Constant58/1 -> Mux3/15
  Constant59/1 -> Mux3/16
  Data Type Conversion3/1 -> Packet/1
  Angle/1 -> Mux3/17
  Speed/1 -> Mux3/18
  Force/1 -> Mux3/19

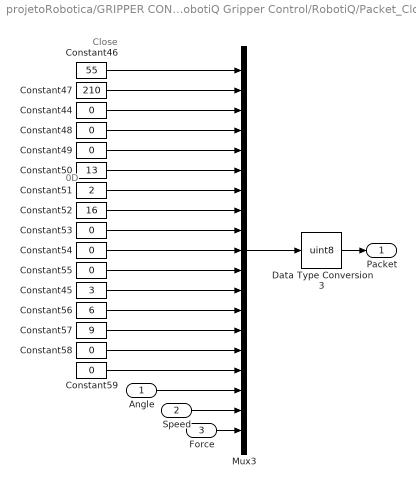
== system projetoRobotica/GRIPPER CONTROL/RobotiQ Gripper Control/RobotiQ/Packet_Close1 ==
  note: Close
  note: 0D
  Angle : Inport
  Speed : Inport  Port=2
  Force : Inport  Port=3
  Constant{44,48..49,53..55,58..59} (8 alike) : Constant  Value=0
  Constant45 : Constant  Value=3
  Constant46 : Constant  Value=55
  Constant47 : Constant  Value=210
  Constant50 : Constant  Value=13
  Constant51 : Constant  Value=2
  Constant52 : Constant  Value=16
  Constant56 : Constant  Value=6
  Constant57 : Constant  Value=9
  Data Type Conversion3 : DataTypeConversion  OutDataTypeStr=uint8
  Mux3 : Mux  Inputs=19
  Packet : Outport
  wires:
  Force/1 -> Mux3/19
  Speed/1 -> Mux3/18
  Angle/1 -> Mux3/17
  Data Type Conversion3/1 -> Packet/1
  Constant59/1 -> Mux3/16
  Constant58/1 -> Mux3/15
  Constant57/1 -> Mux3/14
  Constant56/1 -> Mux3/13
  Constant47/1 -> Mux3/2
  Constant46/1 -> Mux3/1
  Constant45/1 -> Mux3/12
  Constant55/1 -> Mux3/11
  Constant54/1 -> Mux3/10
  Constant53/1 -> Mux3/9
  Constant52/1 -> Mux3/8
  Constant51/1 -> Mux3/7
  Constant50/1 -> Mux3/6
  Constant49/1 -> Mux3/5
  Constant48/1 -> Mux3/4
  Constant44/1 -> Mux3/3
  Mux3/1 -> Data Type Conversion3/1

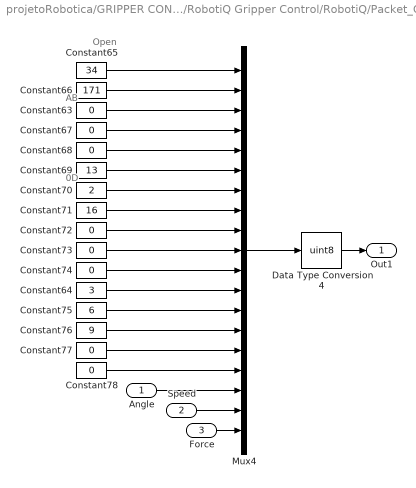
== system projetoRobotica/GRIPPER CONTROL/RobotiQ Gripper Control/RobotiQ/Packet_Open ==
  note: AB
  note: 0D
  note: Open
  Angle : Inport
  Speed : Inport  Port=2
  Force : Inport  Port=3
  Constant{63,67..68,72..74,77..78} (8 alike) : Constant  Value=0
  Constant64 : Constant  Value=3
  Constant65 : Constant  Value=34
  Constant66 : Constant  Value=171
  Constant69 : Constant  Value=13
  Constant70 : Constant  Value=2
  Constant71 : Constant  Value=16
  Constant75 : Constant  Value=6
  Constant76 : Constant  Value=9
  Data Type Conversion4 : DataTypeConversion  OutDataTypeStr=uint8
  Mux4 : Mux  Inputs=19
  Out1 : Outport
  wires:
  Mux4/1 -> Data Type Conversion4/1
  Constant63/1 -> Mux4/3
  Constant67/1 -> Mux4/4
  Constant68/1 -> Mux4/5
  Constant69/1 -> Mux4/6
  Constant70/1 -> Mux4/7
  Constant71/1 -> Mux4/8
  Constant72/1 -> Mux4/9
  Constant73/1 -> Mux4/10
  Constant74/1 -> Mux4/11
  Constant64/1 -> Mux4/12
  Constant65/1 -> Mux4/1
  Constant66/1 -> Mux4/2
  Constant75/1 -> Mux4/13
  Constant76/1 -> Mux4/14
  Constant77/1 -> Mux4/15
  Constant78/1 -> Mux4/16
  Data Type Conversion4/1 -> Out1/1
  Angle/1 -> Mux4/17
  Speed/1 -> Mux4/18
  Force/1 -> Mux4/19

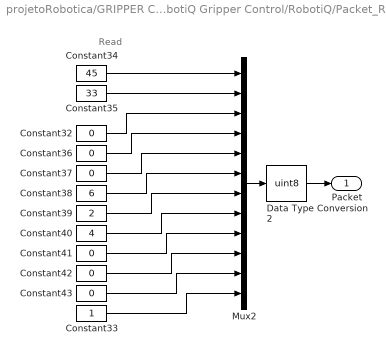
== system projetoRobotica/GRIPPER CONTROL/RobotiQ Gripper Control/RobotiQ/Packet_Read ==
  note: Read
  Constant{32,36..37,41..43} (6 alike) : Constant  Value=0
  Constant33 : Constant
  Constant34 : Constant  Value=45
  Constant35 : Constant  Value=33
  Constant38 : Constant  Value=6
  Constant39 : Constant  Value=2
  Constant40 : Constant  Value=4
  Data Type Conversion2 : DataTypeConversion  OutDataTypeStr=uint8
  Mux2 : Mux  Inputs=12
  Packet : Outport
  wires:
  Mux2/1 -> Data Type Conversion2/1
  Constant32/1 -> Mux2/3
  Constant36/1 -> Mux2/4
  Constant37/1 -> Mux2/5
  Constant38/1 -> Mux2/6
  Constant39/1 -> Mux2/7
  Constant40/1 -> Mux2/8
  Constant41/1 -> Mux2/9
  Constant42/1 -> Mux2/10
  Constant43/1 -> Mux2/11
  Constant33/1 -> Mux2/12
  Constant34/1 -> Mux2/1
  Constant35/1 -> Mux2/2
  Data Type Conversion2/1 -> Packet/1

== matlab function projetoRobotica/MATLAB Function ==
  data: u input; y output
function y  = fcn(u)

if all(u == [0, 0, 0, 0, 0, 0, 0 ]')
    y = [0, 0, -pi/2, 0, 0, 0, 0]';
else
    y = u;
end

== matlab function projetoRobotica/Denso Controller/Scope Indexing Subsystem The first two inputs are the vectors to be compared. The third input is an index to define the elements in each vector to be compared./Dynamic Router1 ==
  data: array input; signal output; index input
function signal = Route(array,index)
signal = array(index);

== matlab function projetoRobotica/Denso Controller/Scope Indexing Subsystem The first two inputs are the vectors to be compared. The third input is an index to define the elements in each vector to be compared./Dynamic Router ==
  data: array input; signal output; index input
function signal = Route(array,index)
signal = array(index);
